simulink model "simulink_aula_1"  (R2022a)
settings: Solver=VariableStepAuto  StartTime=0.0  StopTime=10.0  RelTol=1e-3
values from neighbouring files (symbols this model uses):
  den1 = [1 2 5]    [Aula_1_Scon.m]
  den2 = [1 1]    [Aula_1_Scon.m]
  num1 = 10    [Aula_1_Scon.m]
  num2 = 1    [Aula_1_Scon.m]
settings Model: NumberOfSteps=10  Creator=caugu  LastModifiedBy=caugu

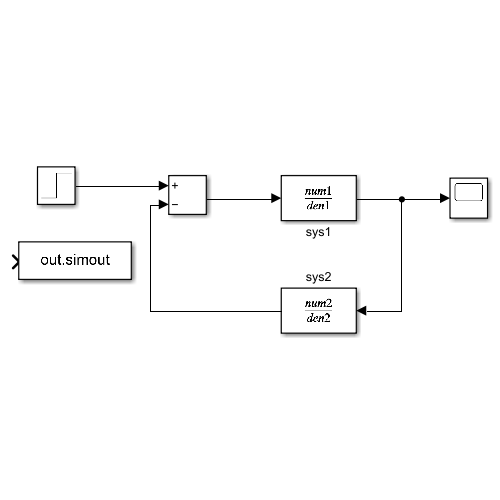
[thumbnail: Simulink's stored preview of the top-level diagram]
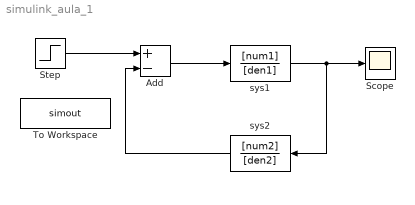
== system simulink_aula_1 ==
  Add : Sum  Inputs=+-
  Scope : Scope
  Step : Step  SampleTime=0
  To Workspace : ToWorkspace  VariableName=simout  SaveFormat=Timeseries  SampleTime=-1
  sys1 : TransferFcn  Numerator=[num1]  Denominator=[den1]
  sys2 : TransferFcn  Numerator=[num2]  Denominator=[den2]
  wires:
  Step/1 -> Add/1
  Add/1 -> sys1/1
  sys1/1 -> sys2/1, Scope/1
  sys2/1 -> Add/2
